simulink model "traffic_light"  (R2017b)
settings: Solver=FixedStepDiscrete  StartTime=0.0  StopTime=10.0  RelTol=1e-3
settings Model: Creator=ibrahim  LastModifiedBy=ibrahim
settings OptimizationCC: DefaultParameterBehavior=Inlined  PassReuseOutputArgsAs=Individual arguments
settings DebuggingCC: ParameterTunabilityLossMsg=error
settings SFSimCC: MATLABDynamicMemAlloc=off
settings RTWCC: SystemTargetFile=ert.tlc  GenCodeOnly=on  TemplateMakefile=ert_default_tmf  GenerateReport=on  IncludeHyperlinkInReport=on  LaunchReport=on  GenerateTraceInfo=on  GenerateTraceReport=on  GenerateTraceReportSl=on  GenerateTraceReportSf=on  GenerateTraceReportEml=on  GenerateWebview=on
settings CodeAppCC: ForceParamTrailComments=on  IgnoreCustomStorageClasses=off  OperatorAnnotations=on  SimulinkDataObjDesc=on  SFDataObjDesc=on  InsertBlockDesc=on
settings ERTTargetCC: TargetLangStandard=C99 (ISO)  GenerateSampleERTMain=on  InlinedParameterPlacement=NonHierarchical  ERTCustomFileTemplate=example_file_process.tlc

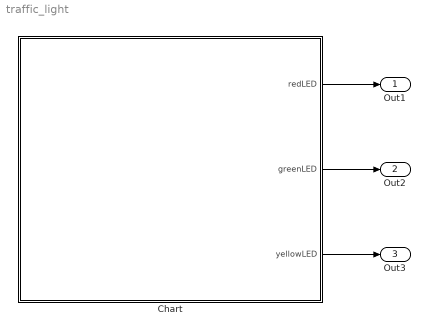
== system traffic_light ==
  Chart : Stateflow chart  TreatAsAtomicUnit=on
  Out1 : Outport
  Out2 : Outport  Port=2
  Out3 : Outport  Port=3
  wires:
  Chart/1(redLED) -> Out1/1
  Chart/2(greenLED) -> Out2/1
  Chart/3(yellowLED) -> Out3/1

== stateflow chart traffic_light/Chart ==
  state LED_RED
    en:
    redLED = 1;
    ex:
    redLED = 0;
  state LED_GREEN
    en:
    greenLED = 1;
    ex:
    greenLED = 0;
  state LED_YELLOW
    en:
    yellowLED = 1;
    ex:
    yellowLED = 0;
  (default) -> (junction 4)
  (junction 4) -> LED_RED
  LED_YELLOW -> LED_RED : {after(200, sec);}
  LED_RED -> LED_GREEN : {after(200, sec);}
  LED_GREEN -> LED_YELLOW : {after(200, sec);}
  data: redLED output; greenLED output; yellowLED output
